simulink model "firefighting_drone"  (R2021b)
settings: Solver=FixedStepAuto  StartTime=0.0  StopTime=80  FixedStep=0.5  RelTol=1e-3
(part 4 of 4)

== system firefighting_drone/Search for Fire/Seaerch-fire/Search7/Move Arm3/Subsystem ==
  Desired Angle : Inport
  Current Angle : Inport  Port=2
  Abs : Abs
  Constant : Constant
  Logical Operator : Logic  Operator=OR  AllPortsSameDT=off  OutDataTypeStr=boolean
  Memory : Memory
  Relational Operator : RelationalOperator  Operator=<=  OutDataTypeStr=boolean  RndMeth=Simplest
  Sum : Sum  Inputs=|+-
  Switch1 : Switch  Criteria=u2 > Threshold
  Out1 : Outport  VectorParamsAs1DForOutWhenUnconnected=off
  Done : Outport  Port=2  VectorParamsAs1DForOutWhenUnconnected=off
  wires:
  Switch1/1 -> Out1/1
  Desired Angle/1 -> Sum/1, Switch1/1
  Current Angle/1 -> Switch1/3, Sum/2
  Sum/1 -> Abs/1
  Abs/1 -> Relational Operator/1
  Constant/1 -> Relational Operator/2
  Relational Operator/1 -> Logical Operator/2
  Logical Operator/1 -> Memory/1, Done/1, Switch1/2
  Memory/1 -> Logical Operator/1

== system firefighting_drone/Search for Fire/Seaerch-fire/Search8/Move Arm1/If Action Subsystem ==
  In1 : Inport
  Action Port : ActionPort  ActionPortLabel=if(u1 > 0)
  Out1 : Outport  VectorParamsAs1DForOutWhenUnconnected=off
  wires:
  In1/1 -> Out1/1

== system firefighting_drone/Search for Fire/Seaerch-fire/Search8/Move Arm1/If Action Subsystem1 ==
  In1 : Inport
  Action Port : ActionPort  ActionPortLabel=else
  Out1 : Outport  VectorParamsAs1DForOutWhenUnconnected=off
  wires:
  In1/1 -> Out1/1

== system firefighting_drone/Search for Fire/Seaerch-fire/Search8/Move Arm1/Subsystem ==
  Desired Angle : Inport
  Current Angle : Inport  Port=2
  Abs : Abs
  Constant : Constant
  Logical Operator : Logic  Operator=OR  AllPortsSameDT=off  OutDataTypeStr=boolean
  Memory : Memory
  Relational Operator : RelationalOperator  Operator=<=  OutDataTypeStr=boolean  RndMeth=Simplest
  Scope : Scope
  Scope1 : Scope
  Sum : Sum  Inputs=|+-
  Switch1 : Switch  Criteria=u2 > Threshold
  Out1 : Outport  VectorParamsAs1DForOutWhenUnconnected=off
  Done : Outport  Port=2  VectorParamsAs1DForOutWhenUnconnected=off
  wires:
  Switch1/1 -> Out1/1
  Desired Angle/1 -> Scope/1, Sum/1, Switch1/1
  Current Angle/1 -> Scope1/1, Switch1/3, Sum/2
  Sum/1 -> Abs/1
  Abs/1 -> Relational Operator/1
  Constant/1 -> Relational Operator/2
  Relational Operator/1 -> Logical Operator/2
  Logical Operator/1 -> Memory/1, Done/1, Switch1/2
  Memory/1 -> Logical Operator/1

== system firefighting_drone/Search for Fire/Seaerch-fire/Search8/Move Arm2/If Action Subsystem ==
  In1 : Inport
  Action Port : ActionPort  ActionPortLabel=if(u1 > 0)
  Out1 : Outport  VectorParamsAs1DForOutWhenUnconnected=off
  wires:
  In1/1 -> Out1/1

== system firefighting_drone/Search for Fire/Seaerch-fire/Search8/Move Arm2/If Action Subsystem1 ==
  In1 : Inport
  Action Port : ActionPort  ActionPortLabel=else
  Out1 : Outport  VectorParamsAs1DForOutWhenUnconnected=off
  wires:
  In1/1 -> Out1/1

== system firefighting_drone/Search for Fire/Seaerch-fire/Search8/Move Arm2/Subsystem ==
  Desired Angle : Inport
  Current Angle : Inport  Port=2
  Abs : Abs
  Constant : Constant
  Logical Operator : Logic  Operator=OR  AllPortsSameDT=off  OutDataTypeStr=boolean
  Memory : Memory
  Relational Operator : RelationalOperator  Operator=<=  OutDataTypeStr=boolean  RndMeth=Simplest
  Sum : Sum  Inputs=|+-
  Switch1 : Switch  Criteria=u2 > Threshold
  Out1 : Outport  VectorParamsAs1DForOutWhenUnconnected=off
  Done : Outport  Port=2  VectorParamsAs1DForOutWhenUnconnected=off
  wires:
  Switch1/1 -> Out1/1
  Desired Angle/1 -> Sum/1, Switch1/1
  Current Angle/1 -> Switch1/3, Sum/2
  Sum/1 -> Abs/1
  Abs/1 -> Relational Operator/1
  Constant/1 -> Relational Operator/2
  Relational Operator/1 -> Logical Operator/2
  Logical Operator/1 -> Memory/1, Done/1, Switch1/2
  Memory/1 -> Logical Operator/1

== system firefighting_drone/Search for Fire/Seaerch-fire/Search8/Move Arm3/If Action Subsystem ==
  In1 : Inport
  Action Port : ActionPort  ActionPortLabel=if(u1 > 0)
  Out1 : Outport  VectorParamsAs1DForOutWhenUnconnected=off
  wires:
  In1/1 -> Out1/1

== system firefighting_drone/Search for Fire/Seaerch-fire/Search8/Move Arm3/If Action Subsystem1 ==
  In1 : Inport
  Action Port : ActionPort  ActionPortLabel=else
  Out1 : Outport  VectorParamsAs1DForOutWhenUnconnected=off
  wires:
  In1/1 -> Out1/1

== system firefighting_drone/Search for Fire/Seaerch-fire/Search8/Move Arm3/Subsystem ==
  Desired Angle : Inport
  Current Angle : Inport  Port=2
  Abs : Abs
  Constant : Constant
  Logical Operator : Logic  Operator=OR  AllPortsSameDT=off  OutDataTypeStr=boolean
  Memory : Memory
  Relational Operator : RelationalOperator  Operator=<=  OutDataTypeStr=boolean  RndMeth=Simplest
  Sum : Sum  Inputs=|+-
  Switch1 : Switch  Criteria=u2 > Threshold
  Out1 : Outport  VectorParamsAs1DForOutWhenUnconnected=off
  Done : Outport  Port=2  VectorParamsAs1DForOutWhenUnconnected=off
  wires:
  Switch1/1 -> Out1/1
  Desired Angle/1 -> Sum/1, Switch1/1
  Current Angle/1 -> Switch1/3, Sum/2
  Sum/1 -> Abs/1
  Abs/1 -> Relational Operator/1
  Constant/1 -> Relational Operator/2
  Relational Operator/1 -> Logical Operator/2
  Logical Operator/1 -> Memory/1, Done/1, Switch1/2
  Memory/1 -> Logical Operator/1

== system firefighting_drone/Search for Fire/Seaerch-fire/Search9/Move Arm1/If Action Subsystem ==
  In1 : Inport
  Action Port : ActionPort  ActionPortLabel=if(u1 > 0)
  Out1 : Outport  VectorParamsAs1DForOutWhenUnconnected=off
  wires:
  In1/1 -> Out1/1

== system firefighting_drone/Search for Fire/Seaerch-fire/Search9/Move Arm1/If Action Subsystem1 ==
  In1 : Inport
  Action Port : ActionPort  ActionPortLabel=else
  Out1 : Outport  VectorParamsAs1DForOutWhenUnconnected=off
  wires:
  In1/1 -> Out1/1

== system firefighting_drone/Search for Fire/Seaerch-fire/Search9/Move Arm1/Subsystem ==
  Desired Angle : Inport
  Current Angle : Inport  Port=2
  Abs : Abs
  Constant : Constant
  Logical Operator : Logic  Operator=OR  AllPortsSameDT=off  OutDataTypeStr=boolean
  Memory : Memory
  Relational Operator : RelationalOperator  Operator=<=  OutDataTypeStr=boolean  RndMeth=Simplest
  Scope : Scope
  Scope1 : Scope
  Sum : Sum  Inputs=|+-
  Switch1 : Switch  Criteria=u2 > Threshold
  Out1 : Outport  VectorParamsAs1DForOutWhenUnconnected=off
  Done : Outport  Port=2  VectorParamsAs1DForOutWhenUnconnected=off
  wires:
  Switch1/1 -> Out1/1
  Desired Angle/1 -> Scope/1, Sum/1, Switch1/1
  Current Angle/1 -> Scope1/1, Switch1/3, Sum/2
  Sum/1 -> Abs/1
  Abs/1 -> Relational Operator/1
  Constant/1 -> Relational Operator/2
  Relational Operator/1 -> Logical Operator/2
  Logical Operator/1 -> Memory/1, Done/1, Switch1/2
  Memory/1 -> Logical Operator/1

== system firefighting_drone/Search for Fire/Seaerch-fire/Search9/Move Arm2/If Action Subsystem ==
  In1 : Inport
  Action Port : ActionPort  ActionPortLabel=if(u1 > 0)
  Out1 : Outport  VectorParamsAs1DForOutWhenUnconnected=off
  wires:
  In1/1 -> Out1/1

== system firefighting_drone/Search for Fire/Seaerch-fire/Search9/Move Arm2/If Action Subsystem1 ==
  In1 : Inport
  Action Port : ActionPort  ActionPortLabel=else
  Out1 : Outport  VectorParamsAs1DForOutWhenUnconnected=off
  wires:
  In1/1 -> Out1/1

== system firefighting_drone/Search for Fire/Seaerch-fire/Search9/Move Arm2/Subsystem ==
  Desired Angle : Inport
  Current Angle : Inport  Port=2
  Abs : Abs
  Constant : Constant
  Logical Operator : Logic  Operator=OR  AllPortsSameDT=off  OutDataTypeStr=boolean
  Memory : Memory
  Relational Operator : RelationalOperator  Operator=<=  OutDataTypeStr=boolean  RndMeth=Simplest
  Sum : Sum  Inputs=|+-
  Switch1 : Switch  Criteria=u2 > Threshold
  Out1 : Outport  VectorParamsAs1DForOutWhenUnconnected=off
  Done : Outport  Port=2  VectorParamsAs1DForOutWhenUnconnected=off
  wires:
  Switch1/1 -> Out1/1
  Desired Angle/1 -> Sum/1, Switch1/1
  Current Angle/1 -> Switch1/3, Sum/2
  Sum/1 -> Abs/1
  Abs/1 -> Relational Operator/1
  Constant/1 -> Relational Operator/2
  Relational Operator/1 -> Logical Operator/2
  Logical Operator/1 -> Memory/1, Done/1, Switch1/2
  Memory/1 -> Logical Operator/1

== system firefighting_drone/Search for Fire/Seaerch-fire/Search9/Move Arm3/If Action Subsystem ==
  In1 : Inport
  Action Port : ActionPort  ActionPortLabel=if(u1 > 0)
  Out1 : Outport  VectorParamsAs1DForOutWhenUnconnected=off
  wires:
  In1/1 -> Out1/1

== system firefighting_drone/Search for Fire/Seaerch-fire/Search9/Move Arm3/If Action Subsystem1 ==
  In1 : Inport
  Action Port : ActionPort  ActionPortLabel=else
  Out1 : Outport  VectorParamsAs1DForOutWhenUnconnected=off
  wires:
  In1/1 -> Out1/1

== system firefighting_drone/Search for Fire/Seaerch-fire/Search9/Move Arm3/Subsystem ==
  Desired Angle : Inport
  Current Angle : Inport  Port=2
  Abs : Abs
  Constant : Constant
  Logical Operator : Logic  Operator=OR  AllPortsSameDT=off  OutDataTypeStr=boolean
  Memory : Memory
  Relational Operator : RelationalOperator  Operator=<=  OutDataTypeStr=boolean  RndMeth=Simplest
  Sum : Sum  Inputs=|+-
  Switch1 : Switch  Criteria=u2 > Threshold
  Out1 : Outport  VectorParamsAs1DForOutWhenUnconnected=off
  Done : Outport  Port=2  VectorParamsAs1DForOutWhenUnconnected=off
  wires:
  Switch1/1 -> Out1/1
  Desired Angle/1 -> Sum/1, Switch1/1
  Current Angle/1 -> Switch1/3, Sum/2
  Sum/1 -> Abs/1
  Abs/1 -> Relational Operator/1
  Constant/1 -> Relational Operator/2
  Relational Operator/1 -> Logical Operator/2
  Logical Operator/1 -> Memory/1, Done/1, Switch1/2
  Memory/1 -> Logical Operator/1
